simulink model "pid_penalty_24a"  (R2024a)
settings: Solver=VariableStepAuto  StartTime=0.0  StopTime=inf  RelTol=1e-3
PreLoadFcn:
  | modellSti = fileparts(which(bdroot));
  | addpath(genpath(fullfile(modellSti, 'mqtt')));
  | addpath(genpath('mqtt'));
libraries: send x3, read x2, init_b x2
settings Model: Creator=eikel  LastModifiedBy=adriaeik

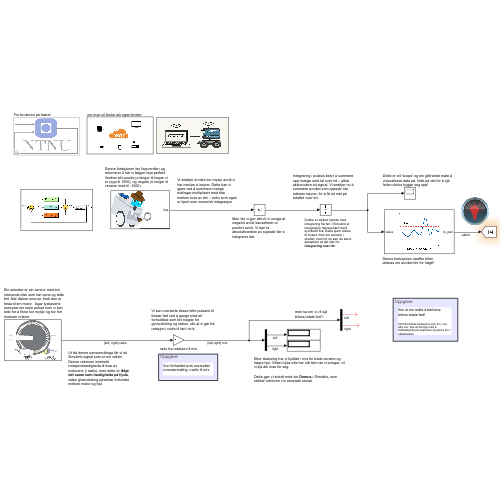
[thumbnail: Simulink's stored preview of the top-level diagram]
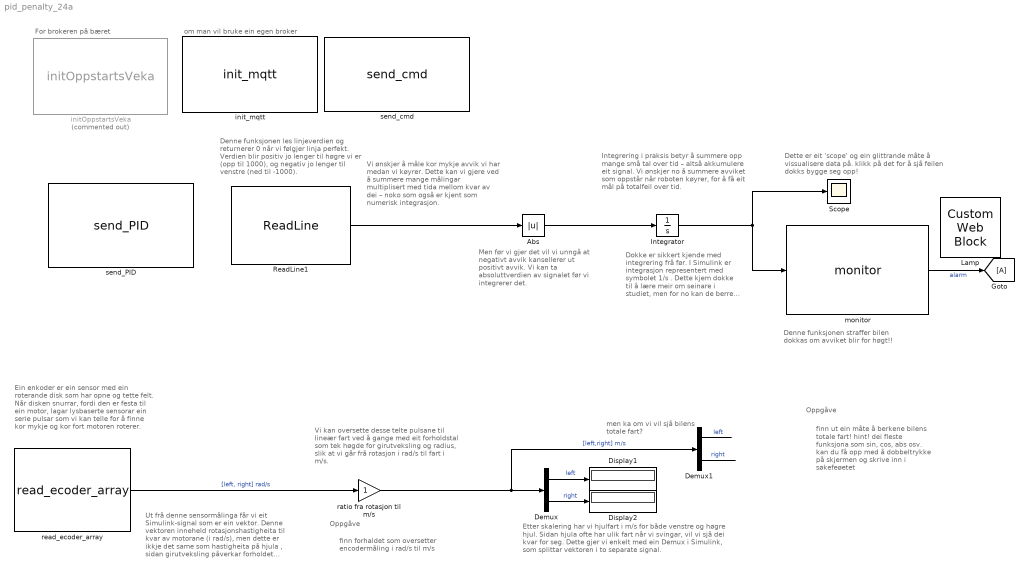
== system pid_penalty_24a ==
  note: om man vil bruke ein egen broker
  note: For brokeren på bæret
  note: Dette er eit 'scope' og ein glittrande måte å vissualisere data på. klikk på det for å sjå feilen dokks bygge seg opp!
  note: Denne funksjonen straffer bilen dokkas om avviket blir for høgt!!
  note: Vi ønskjer å måle kor mykje avvik vi har medan vi køyrer. Dette kan vi gjere ved å summere mange målingar multiplisert med tida mellom kvar av dei – noko som også er kjent som numerisk integrasjon.
  note: Denne funksjonen les linjeverdien og returnerer 0 når vi følgjer linja perfekt. Verdien blir positiv jo lenger til høgre vi er (opp til 1000), og negativ jo lenger til venstre (ned til -1000).
  note: Men før vi gjer det vil vi unngå at negativt avvik kansellerer ut positivt avvik. Vi kan ta absoluttverdien av signalet før vi integrerer det.
  note: Integrering i praksis betyr å summere opp mange små tal over tid – altså akkumulere eit signal. Vi ønskjer no å summere avviket som oppstår når roboten køyrer, for å få eit mål på totalfeil over tid.
  note: Dokke er sikkert kjende med integrering frå før. I Simulink er integrasjon representert med symbolet 1/s . Dette kjem dokke til å lære meir om seinare i studiet, men for no kan de berre akseptere at det står for integrering over tid .
  note: men ka om vi vil sjå bilens totale fart?
  note: Etter skalering har vi hjulfart i m/s for både venstre og høgre hjul. Sidan hjula ofte har ulik fart når vi svingar, vil vi sjå dei kvar for seg.
      | Dette gjer vi enkelt med ein Demux i Simulink, som splittar vektoren i to separate signal.
  note: Oppgåve
  note: finn forhaldet som oversetter encodermåling i rad/s til m/s
  note: Ut frå denne sensormålinga får vi eit Simulink-signal som er ein vektor. Denne vektoren inneheld rotasjonshastigheita til kvar av motorane (i rad/s), men dette er ikkje det same som hastigheita på hjula , sidan girutveksling påverkar forholdet mellom motor og hjul.
  note: Vi kan oversette desse telte pulsane til lineær fart ved å gange med eit forholdstal som tek høgde for girutveksling og radius, slik at vi går frå rotasjon i rad/s til fart i m/s.
  note: Ein enkoder er ein sensor med ein roterande disk som har opne og tette felt. Når disken snurrar, fordi den er festa til ein motor, lagar lysbaserte sensorar ein serie pulsar som vi kan telle for å finne kor mykje og kor fort motoren roterer.
  note: Oppgåve
  note: finn ut ein måte å berkene bilens totale fart!
      |
      | hint! dei fleste funksjona som sin, cos, abs osv. kan du få opp med å dobbeltrykke på skjermen og skrive inn i søkefeøetet
  Abs : Abs  SaturateOnIntegerOverflow=off
  Demux : Demux  Outputs=2
  Demux1 : Demux  Outputs=2
  Display1 : Display
  Display2 : Display
  Goto : Goto
  Integrator : Integrator
  Lamp : CustomWebBlock  LabelPosition=Hide  ShowInitialText=on  Configuration="{\"components\":[{\"name\":\"BackgroundImageComponent\",\"settings\":{\"image\":{\"size\":[150,150],\"src\":\"data:image\\/svg+xml;base64,PHN2ZyB4bWxucz0iaHR0cDovL3d3dy53My5vcmcvMjAwMC9zdmciIHhtbG5zOnhsaW5rPSJodHRwOi8vd3d3LnczLm9yZy8xOTk5L3hsaW5rIiB2aWV3Qm94PSIwIDAgNTAwIDUwMCI+PGRlZnM+PHN0eWxlPi5he2ZpbGw6dXJsKCNhKTt9LmJ7ZmlsbDp1cmwoI2IpO30uY3tmaWxsOnVybCgjYyk7fTwvc3R5bGU+PHJhZGlhbEdyYWRpZW50IGlkPSJhIiBjeD0iMjgzLjg0IiBjeT0iLTQ2Ni4zNyIgcj0iMzc1Ljc1IiBncmFkaWVudFRyYW5zZm9ybT0ibWF0cml4KDEuMzksIDAsIDAsIC0xLjM5LCAtMTUzLjU2LCAtNjQ0LjA4KSIg ...(+2088 chars)\",\"srcOrientation\":\"Right\"},\"position\":[0,0,1,1],\"scaleMode\":\"0\"}},{\"name\":\"LampStateComponent\",\"settings\":{\"position\":[0,0,1,1],\"states\":[{\"icon\":{\"customSrc\":\"data:image\\/svg+xml;base64,PHN2ZyBpZD0iTGF5ZXJfMSIgZGF0YS1uYW1lPSJMYXllciAxIiB4bWxucz0iaHR0cDovL3d3dy53My5vcmcvMjAwMC9zdmciIHZpZXdCb3g9IjAgMCA0MTEgNDU4Ij48ZGVmcz48c3R5bGU+LmNscy0xe2ZpbGw6I2ZkZjhjMTt9LmNscy0ye2ZpbGw6I2ZlZTEwMDt9LmNscy0ze2ZpbGw6IzIzMWYyMDt9LmNscy00e2ZpbGw6I2EwOWY5Zjt9LmNscy00LC5jbHMtNSwuY2xzLTZ7c3Ryb2tlOiMyMzFmMjA7c3Ryb2tlLW1pdGVybGltaXQ6MTA7fS5jbHMtNXtmaWxsOiNmZmY7fS5jbHMtNntmaWxsOm5vbmU7fTwvc3R5bGU+PC9kZWZz ...(+5168 chars)\",\"id\":-1,\"srcOrientation\":\"Right\",\"type\":\"custom\"},\"iconScale\":0.8,\"metadata\":{},\"overlayType\":\"intersect\",\"shape\":{\"color\":[0.725,0,0],\"opacity\":1,\"position\":[0.1,0.1,0.8,0.8],\"type\":\"ellipse\"},\"value\":[]},{\"icon\":{\"customSrc\":\"data:image\\/svg+xml;base64,PHN2ZyBpZD0iTGF5ZXJfMSIgZGF0YS1uYW1lPSJMYXllciAxIiB4bWxucz0iaHR0cDovL3d3dy53My5vcmcvMjAwMC9zdmciIHZpZXdCb3g9IjAgMCA0MTEgNDU4Ij48ZGVmcz48c3R5bGU+LmNscy0xe2ZpbGw6I2ZkZjhjMTt9LmNscy0ye2ZpbGw6I2ZlZTEwMDt9LmNscy0ze2ZpbGw6IzIzMWYyMDt9LmNscy00e2ZpbGw6I2EwOWY5Zjt9LmNscy00LC5jbHMtNSwuY2xzLTZ7c3Ryb2tlOiMyMzFmMjA7c3Ryb2tlLW1pdGVybGltaXQ6MTA7fS5jbHMtNXtmaWxsOiNmZmY7fS5jbHMtNntmaWxsOm5vbmU7fTwvc3R5bGU+PC9kZWZz ...(+5168 chars)\",\"id\":-1,\"srcOrientation\":\"Right\",\"type\":\"custom\"},\"iconScale\":0.8,\"metadata\":{\"useDefaults\":{\"customIcon\":true,\"icon\":true,\"overlayType\":true,\"shape\":true,\"sizeAndPosition\":true}},\"overlayType\":\"intersect\",\"shape\":{\"color\":[1,1,1],\"opacity\":1,\"position\":[0.1,0.1,0.8,0.8],\"type\":\"ellipse\"},\"value\":\"0\"},{\"icon\":{\"customSrc\":\"data:image\\/svg+xml;base64,PHN2ZyBpZD0iTGF5ZXJfMSIgZGF0YS1uYW1lPSJMYXllciAxIiB4bWxucz0iaHR0cDovL3d3dy53My5vcmcvMjAwMC9zdmciIHZpZXdCb3g9IjAgMCA0MTEgNDU4Ij48ZGVmcz48c3R5bGU+LmNscy0xe2ZpbGw6I2ZkZjhjMTt9LmNscy0ye2ZpbGw6I2ZlZTEwMDt9LmNscy0ze2ZpbGw6IzIzMWYyMDt9LmNscy00e2ZpbGw6I2EwOWY5Zjt9LmNscy00LC5jbHMtNSwuY2xzLTZ7c3Ryb2tlOiMyMzFmMjA7c3Ryb2tlLW1pdGVybGltaXQ6MTA7fS5jbHMtNXtmaWxsOiNmZmY7fS5jbHMtNntmaWxsOm5vbmU7fTwvc3R5bGU+PC9kZWZz ...(+5168 chars)\",\"id\":-1,\"srcOrientation\":\"Right\",\"type\":\"custom\"},\"iconScale\":0.8,\"metadata\":{\"useDefaults\":{\"customIcon\":true,\"icon\":true,\"overlayType\":true,\"shape\":true,\"sizeAndPosition\":true}},\"overlayType\":\"intersect\",\"shape\":{\"color\":[1,0,0],\"opacity\":1,\"position\":[0.1,0.1,0.8,0.8],\"type\":\"ellipse\"},\"value\":\"1\"}],\"valueType\":\"discrete\"}},{\"name\":\"ForegroundImageComponent\",\"settings\":{\"image\":{\"size\":[150,150],\"src\":\"data:image\\/svg+xml;base64,PHN2ZyB4bWxucz0iaHR0cDovL3d3dy53My5vcmcvMjAwMC9zdmciIHhtbG5zOnhsaW5rPSJodHRwOi8vd3d3LnczLm9yZy8xOTk5L3hsaW5rIiB2aWV3Qm94PSIwIDAgNTAwIDUwMCI+PGRlZnM+PHN0eWxlPi5he2ZpbGw6dXJsKCNhKTt9PC9zdHlsZT48bGluZWFyR3JhZGllbnQgaWQ9ImEiIHgxPSIxNzMuMDUiIHkxPSItNjI3Ljc4IiB4Mj0iMTczLjA1IiB5Mj0iLTUyMi40MyIgZ3JhZGllbnRUcmFuc2Zvcm09Im1hdHJpeCgxLjI5LCAwLCAwLCAtMS4zMywgMjcuMTMsIC02MjguMzEpIiBncmFkaWVudFVuaXRzPSJ1c2VyU3BhY2VPblVzZSI+PHN0b3Agb2Zmc2V0PSIwIiBzdG9wLWNvbG9yPSIjZmZmIiBzdG9wLW9wYWNpdHk9IjAuMjUiLz48c3RvcCBvZmZzZXQ9IjEiIHN0b3AtY29sb3I9IiNmZmYiIHN0b3Atb3BhY2l0eT0iMCIvPjwvbGluZWFyR3JhZGllbnQ+PC9kZWZzPjxwYXRoIGNsYXNzPSJhIiBkPSJNNDI5LjMsMTkwLjY2QzQwMi40NSwxMTQuNTEsMzMyLjY3LDYwLjE3LDI1MC44NSw2MC4xN2MtODMuNDMsMC0xNTQuMjgsNTYuNDItMTc5Ljk1LDEzNSwxNS4zNCwzOSw4OC4xMSw3LDE3Ny4wNyw3QzM0MCwyMDIuMDgsNDE3LjI2LDIzNi40Niw0MjkuMywxOTAuNjZaIi8+PC9zdmc+\",\"srcOrientation\":\"Right\"},\"isForeground\":1,\"position\":[0,0,1,1],\"scaleMode\":\"0\"}}],\"settings\":{\"BindingType\":\"signal\",\"aspectRatio\":1.032258064516129,\"backgroundColor\":[0,0,0],\"backgroundOffset\":0.14,\"backgroundOpacity\":1,\"blockOrientation\":\"Right\",\"fixedAspectRatio\":\"on\",\"showBackgroundColor\":false,\"value\":0,\"version\":\"R2023a\"},\"type\":\"Lamp\"}"  StateValueType=Discrete  Icon=Custom
  ReadLine1 : read/ReadLine
  Scope : Scope
  initOppstartsVeka : init_b/initOppstartsVeka  Commented=on  carID=14
  init_mqtt : init_b/init_mqtt  carID=14  brokerVal='localhost'  portVal='1883'  userVal=''  passVal=''
  monitor : send/monitor
  ratio fra rotasjon til m/s : Gain
  read_ecoder_array : read/read_ecoder_array
  send_PID : send/send_PID  kp=0  ki=0  kd=0
  send_cmd : send/send_cmd  cmd=Start
  wires:
  ReadLine1/1 -> Abs/1
  read_ecoder_array/1 -> ratio fra rotasjon til m/s/1  "[left, right] rad/s"
  ratio fra rotasjon til m/s/1 -> Demux1/1, Demux/1  "[left,right] m/s"
  Demux/1 -> Display1/1  "left"
  Demux/2 -> Display2/1  "right"
  Integrator/1 -> monitor/1, Scope/1
  Abs/1 -> Integrator/1
  monitor/1 -> Goto/1  "alarm"
  Demux1/1 -> ?  "left"
  Demux1/2 -> ?  "right"
